simulink model "sourceLocalization3"  (R2020a)
settings: Solver=VariableStepAuto  StartTime=0.0  StopTime=inf  RelTol=1e-3
model workspace (MAT data in the model file):
  VADThreshold = 0.85
  frameLength = 10000
  fs = 44100
undefined symbols (not defined in the file or in its folder): phased
libraries: dspnetwork x5, dspsrcs4 x3, dspvision x3, phaseddoalib x3, audiomeasurements x3, simulink x1
settings Model: OrderedModelArguments=off  Creator=GH  LastModifiedBy=GH
settings DebuggingCC: UnderSpecifiedDimensionMsg=warning

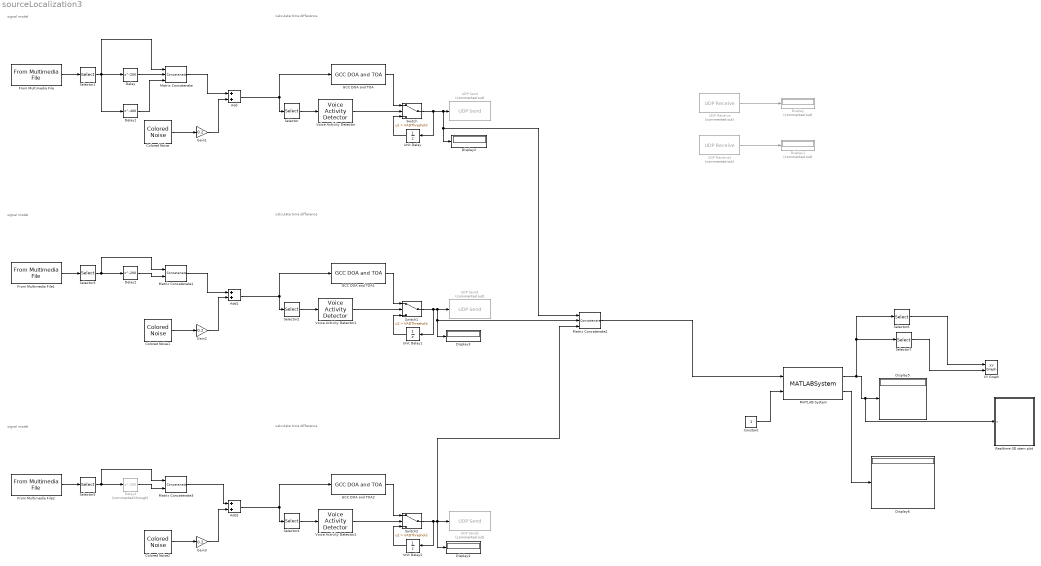
== system sourceLocalization3 ==
  note: calculate time difference
  note: signal model
  note: signal model
  note: calculate time difference
  note: calculate time difference
  note: signal model
  Add : Sum
  Add1 : Sum
  Add2 : Sum
  Colored Noise : dspsrcs4/Colored Noise  Color=pink  InverseFrequencyPower=1  BoundedOutput=on  NumChannels=3  OutputDataType=double  SamplesPerFrame=frameLength  SampleTime=1/fs  RandomStream=mt19937ar with seed  Seed=67  SimulateUsing=Interpreted execution
      settings: SourceProductBaseCode=DS
  Colored Noise1 : dspsrcs4/Colored Noise  Color=pink  InverseFrequencyPower=1  BoundedOutput=on  NumChannels=2  OutputDataType=double  SamplesPerFrame=frameLength  SampleTime=1/fs  RandomStream=mt19937ar with seed  Seed=67  SimulateUsing=Interpreted execution
      settings: SourceProductBaseCode=DS
  Colored Noise2 : dspsrcs4/Colored Noise  Color=pink  InverseFrequencyPower=1  BoundedOutput=on  NumChannels=2  OutputDataType=double  SamplesPerFrame=frameLength  SampleTime=1/fs  RandomStream=mt19937ar with seed  Seed=67  SimulateUsing=Interpreted execution
      settings: SourceProductBaseCode=DS
  Constant : Constant
  Delay : Delay  DelayLength=200  InputProcessing=Columns as channels (frame based)  UseCircularBuffer=on
  Delay1 : Delay  DelayLength=400  InputProcessing=Columns as channels (frame based)  UseCircularBuffer=on
  Delay2 : Delay  DelayLength=200  InputProcessing=Columns as channels (frame based)  UseCircularBuffer=on
  Delay4 : Delay  Commented=through  DelayLength=200  InputProcessing=Columns as channels (frame based)  UseCircularBuffer=on
  Display : Display  Commented=on
  Display1 : Display  Commented=on
  Display{2..6} (5 alike) : Display
  From Multimedia File : dspvision/From Multimedia File  inputFilename=D:\Files\Research\1a 其他\测试用音频\美谈不美repair.wav  readRange=[1 Inf]  loop=on  numPlays=inf  outputStreams=Audio only  videoDataType=single  audioDataType=double  inheritSampleTime=on  userDefinedSampleTime=1/30  noAudioOutput=off  isIntensityVideo=off  fourcc=RGB  colorVideoFormat=Separate color signals  outputEOF=off  dataOrg=Column-major  audioFrameSize=frameLength  computeAudioFrameSize=off  outSamplingMode=Sample based
  From Multimedia File1 : dspvision/From Multimedia File  inputFilename=D:\Files\Research\1a 其他\测试用音频\美谈不美repair.wav  readRange=[1 Inf]  loop=on  numPlays=inf  outputStreams=Audio only  videoDataType=single  audioDataType=double  inheritSampleTime=on  userDefinedSampleTime=1/30  noAudioOutput=off  isIntensityVideo=off  fourcc=RGB  colorVideoFormat=Separate color signals  outputEOF=off  dataOrg=Column-major  audioFrameSize=frameLength  computeAudioFrameSize=off  outSamplingMode=Sample based
  From Multimedia File2 : dspvision/From Multimedia File  inputFilename=D:\Files\Research\1a 其他\测试用音频\美谈不美repair.wav  readRange=[1 Inf]  loop=on  numPlays=inf  outputStreams=Audio only  videoDataType=single  audioDataType=double  inheritSampleTime=on  userDefinedSampleTime=1/30  noAudioOutput=off  isIntensityVideo=off  fourcc=RGB  colorVideoFormat=Separate color signals  outputEOF=off  dataOrg=Column-major  audioFrameSize=frameLength  computeAudioFrameSize=off  outSamplingMode=Sample based
  GCC DOA and TOA : phaseddoalib/GCC DOA and TOA  PropagationSpeed=300  SampleRateFromInputCheckbox=on  SampleRate=1e6  SensorPairSource=Auto  SensorPair=[ 2; 1 ]  CorrelationOutputPort=off  DelayOutputPort=off  SimulateUsing=Interpreted execution  SensorArray=phased.ULA('NumElements',3,'ElementSpacing',200/44100/sind(30)*300,'ArrayAxis','y','Element',phased.OmnidirectionalMicrophoneElement('BackBaffled',false))
      settings: SourceProductBaseCode=AR
  GCC DOA and TOA1 : phaseddoalib/GCC DOA and TOA  PropagationSpeed=300  SampleRateFromInputCheckbox=on  SampleRate=1e6  SensorPairSource=Auto  SensorPair=[ 2; 1 ]  CorrelationOutputPort=off  DelayOutputPort=off  SimulateUsing=Interpreted execution  SensorArray=phased.ULA('NumElements',2,'ElementSpacing',200/44100/sind(30)*300,'ArrayAxis','y','Element',phased.OmnidirectionalMicrophoneElement('BackBaffled',false))
      settings: SourceProductBaseCode=AR
  GCC DOA and TOA2 : phaseddoalib/GCC DOA and TOA  PropagationSpeed=300  SampleRateFromInputCheckbox=on  SampleRate=1e6  SensorPairSource=Auto  SensorPair=[ 2; 1 ]  CorrelationOutputPort=off  DelayOutputPort=off  SimulateUsing=Interpreted execution  SensorArray=phased.ULA('NumElements',2,'ElementSpacing',200/44100/sind(45)*300,'ArrayAxis','y','Element',phased.OmnidirectionalMicrophoneElement('BackBaffled',false))
      settings: SourceProductBaseCode=AR
  Gain1 : Gain  Gain=0.2
  Gain2 : Gain  Gain=0.2
  Gain3 : Gain  Gain=0.2
  MATLAB System : MATLABSystem  System=getSourcePosition  arrayPos=[0 0 1;-1 1 1;1 1 1].'  arrayAxis=[2 0 0;0 1 0;0 0 1].'  maxStepLength=0.2  SimulateUsing=Interpreted execution
      mask Type: getSourcePosition
      mask Display:
      | disp('getSourcePosition');
      | port_label('input',1,'aoa');
      | port_label('input',2,'calFlag');
      | port_label('output',1,'sourcePosition');
      | port_label('output',2,'dr');
  Matrix Concatenate : Concatenate  NumInputs=3  Mode=Multidimensional array  ConcatenateDimension=2
  Matrix Concatenate1 : Concatenate  Mode=Multidimensional array  ConcatenateDimension=2
  Matrix Concatenate2 : Concatenate  NumInputs=3  Mode=Multidimensional array  ConcatenateDimension=2
  Matrix Concatenate3 : Concatenate  Mode=Multidimensional array  ConcatenateDimension=2
  Realtime-3D stem plot : MATLAB Function  TreatAsAtomicUnit=on
  Selector{,1..5} (6 alike) : Selector  NumberOfDimensions=2  InputPortWidth=3  IndexOptions=Select all,Index vector (dialog)  Indices=[1 3],1  OutputSizes=1,1
  Selector6 : Selector  NumberOfDimensions=2  InputPortWidth=3  IndexOptions=Index vector (dialog),Select all  Indices=1,[1 2]  OutputSizes=1,1
  Selector7 : Selector  NumberOfDimensions=2  InputPortWidth=3  IndexOptions=Index vector (dialog),Select all  Indices=2,[1 2]  OutputSizes=1,1
  Switch : Switch  Criteria=u2 > Threshold  Threshold=VADThreshold
  Switch1 : Switch  Criteria=u2 > Threshold  Threshold=VADThreshold
  Switch2 : Switch  Criteria=u2 > Threshold  Threshold=VADThreshold
  UDP Receive : dspnetwork/UDP Receive  Commented=on  localURL='0.0.0.0'  localPort=23450  remoteURL='0.0.0.0'  remotePort=-1  recvBufferSize=8192  dims=255  signalDatatype=double  isComplex=off  isVarSize=on  showBlockingTime=off  blockingTime=0  sampletime=frameLength/fs  blockPlatform=[]
  UDP Receive1 : dspnetwork/UDP Receive  Commented=on  localURL='0.0.0.0'  localPort=23451  remoteURL='0.0.0.0'  remotePort=-1  recvBufferSize=8192  dims=255  signalDatatype=double  isComplex=off  isVarSize=on  showBlockingTime=off  blockingTime=0  sampletime=frameLength/fs  blockPlatform=[]
  UDP Send : dspnetwork/UDP Send  Commented=on  remoteURL='127.0.0.1'  remotePort=23450  localURL='0.0.0.0'  localPortSource=Automatically determine  localPort=-1  sendBufferSize=8192  sampletime=-1  blockPlatform=[]  separateLengthPort=0
  UDP Send1 : dspnetwork/UDP Send  Commented=on  remoteURL='127.0.0.1'  remotePort=23451  localURL='0.0.0.0'  localPortSource=Automatically determine  localPort=-1  sendBufferSize=8192  sampletime=-1  blockPlatform=[]  separateLengthPort=0
  UDP Send2 : dspnetwork/UDP Send  Commented=on  remoteURL='127.0.0.1'  remotePort=23452  localURL='0.0.0.0'  localPortSource=Automatically determine  localPort=-1  sendBufferSize=8192  sampletime=-1  blockPlatform=[]  separateLengthPort=0
  Unit Delay : UnitDelay  InputProcessing=Columns as channels (frame based)  SampleTime=-1  HasFrameUpgradeWarning=on
  Unit Delay1 : UnitDelay  InputProcessing=Columns as channels (frame based)  SampleTime=-1  HasFrameUpgradeWarning=on
  Unit Delay2 : UnitDelay  InputProcessing=Columns as channels (frame based)  SampleTime=-1  HasFrameUpgradeWarning=on
  Voice Activity Detector : audiomeasurements/Voice Activity Detector  InputDomain=Time  Window=Hann  SidelobeAttenuation=60  InheritFFTLength=on  FFTLength=1024  SilenceToSpeechProbabilityPort=off  SilenceToSpeechProbability=0.2  SpeechToSilenceProbabilityPort=off  SpeechToSilenceProbability=0.1  OutputNoiseVariance=off  SimulateUsing=Code generation
      settings: SourceProductBaseCode=AU
  Voice Activity Detector1 : audiomeasurements/Voice Activity Detector  InputDomain=Time  Window=Hann  SidelobeAttenuation=60  InheritFFTLength=on  FFTLength=1024  SilenceToSpeechProbabilityPort=off  SilenceToSpeechProbability=0.2  SpeechToSilenceProbabilityPort=off  SpeechToSilenceProbability=0.1  OutputNoiseVariance=off  SimulateUsing=Code generation
      settings: SourceProductBaseCode=AU
  Voice Activity Detector2 : audiomeasurements/Voice Activity Detector  InputDomain=Time  Window=Hann  SidelobeAttenuation=60  InheritFFTLength=on  FFTLength=1024  SilenceToSpeechProbabilityPort=off  SilenceToSpeechProbability=0.2  SpeechToSilenceProbabilityPort=off  SpeechToSilenceProbability=0.1  OutputNoiseVariance=off  SimulateUsing=Code generation
      settings: SourceProductBaseCode=AU
  XY Graph : simulink/Sinks/XY Graph  xmin=-1  xmax=1  ymin=-1  ymax=1  st=-1
  wires:
  From Multimedia File/1 -> Selector1/1
  Delay/1 -> Matrix Concatenate/2
  Delay1/1 -> Matrix Concatenate/3
  GCC DOA and TOA/1 -> Switch/1
  Add/1 -> GCC DOA and TOA/1, Selector/1
  Voice Activity Detector/1 -> Switch/2
  Switch/1 -> Matrix Concatenate2/1, Display2/1, UDP Send/1, Unit Delay/1
  Unit Delay/1 -> Switch/3
  Selector1/1 -> Matrix Concatenate/1, Delay1/1, Delay/1
  Colored Noise/1 -> Gain1/1
  Matrix Concatenate/1 -> Add/1
  Gain1/1 -> Add/2
  Selector/1 -> Voice Activity Detector/1
  UDP Receive/1 -> Display/1
  Matrix Concatenate1/1 -> Add1/1
  Selector3/1 -> Matrix Concatenate1/1, Delay2/1
  Gain2/1 -> Add1/2
  Selector2/1 -> Voice Activity Detector1/1
  Delay2/1 -> Matrix Concatenate1/2
  Colored Noise1/1 -> Gain2/1
  Voice Activity Detector1/1 -> Switch1/2
  Unit Delay1/1 -> Switch1/3
  Switch1/1 -> UDP Send1/1, Display3/1, Matrix Concatenate2/2, Unit Delay1/1
  Add1/1 -> GCC DOA and TOA1/1, Selector2/1
  From Multimedia File1/1 -> Selector3/1
  GCC DOA and TOA1/1 -> Switch1/1
  UDP Receive1/1 -> Display1/1
  Voice Activity Detector2/1 -> Switch2/2
  Delay4/1 -> Matrix Concatenate3/2
  Selector5/1 -> Matrix Concatenate3/1, Delay4/1
  Matrix Concatenate3/1 -> Add2/1
  Unit Delay2/1 -> Switch2/3
  From Multimedia File2/1 -> Selector5/1
  GCC DOA and TOA2/1 -> Switch2/1
  Switch2/1 -> Matrix Concatenate2/3, UDP Send2/1, Display4/1, Unit Delay2/1
  Selector4/1 -> Voice Activity Detector2/1
  Gain3/1 -> Add2/2
  Colored Noise2/1 -> Gain3/1
  Add2/1 -> GCC DOA and TOA2/1, Selector4/1
  MATLAB System/1 -> Selector7/1, Selector6/1, Realtime-3D stem plot/1(x), Display5/1
  Constant/1 -> MATLAB System/2
  MATLAB System/2 -> Display6/1
  Matrix Concatenate2/1 -> MATLAB System/1
  Selector6/1 -> XY Graph/1
  Selector7/1 -> XY Graph/2

== matlab function sourceLocalization3/Realtime-3D stem plot ==
  data: x input
function  fcn(x)
figure(1);
% hold on;
grid on;
coder.extrinsic('stem3');
stem3(x(1), x(2), x(3));
xlim([-1 1]);xlabel(sprintf('x: %f', x(1)));
ylim([-1 1]);ylabel(sprintf('y: %f', x(2)));
zlim([0 2]);zlabel(sprintf('z: %f', x(3)));
view([45 45]);
